simulink model "AircraftModelAdam"  (R2025b)
settings: Solver=VariableStepAuto  StartTime=0.0  StopTime=10  RelTol=1e-3
values from neighbouring files (symbols this model uses):
  forceConstants = [m; g]    [RunAircraftModel_AdamForceMomentVersion.m]
  maxAileronDeflection = 25*(pi/180)    (= 0.436332312999)    [RunAircraftModel_AdamForceMomentVersion.m]
  maxElevatorDeflection = 10*(pi/180)    (= 0.174532925199)    [RunAircraftModel_AdamForceMomentVersion.m]
  maxRudderDeflection = 30*(pi/180)    (= 0.523598775598)    [RunAircraftModel_AdamForceMomentVersion.m]
  momentConstants = [Jx; Jy; Jz; Jxz; Gamma]    [RunAircraftModel_AdamForceMomentVersion.m]
  U0 = 84.9905    [RunAircraftModel_AdamForceMomentVersion.m]
libraries: aerolibfltsims x2, aerolibanimutils x1
settings Model: Creator=Reza  LastModifiedBy=adaml
settings OptimizationCC: ReuseModelBlockBuffer=off
settings DebuggingCC: UnconnectedInputMsg=warning  UnconnectedOutputMsg=warning  UnconnectedLineMsg=warning
settings ModelReferenceCC: EnableRefExpFcnMdlSchedulingChecks=on
settings RTWCC: GPUComputeCapability=3.5  DLArmComputeVersion=19.05
settings SimscapeCC: SimscapeLogDecimation=1  SimscapeLogDataHistory=5000

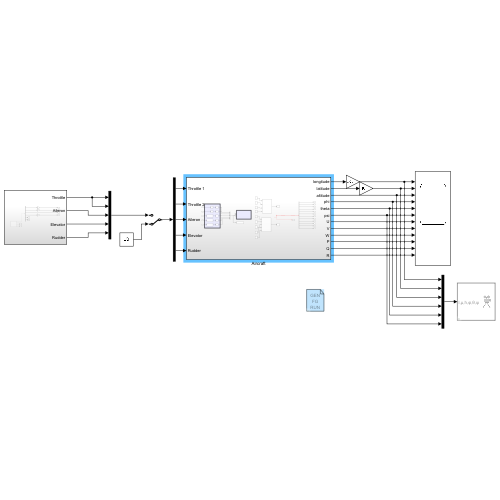
[thumbnail: Simulink's stored preview of the top-level diagram]
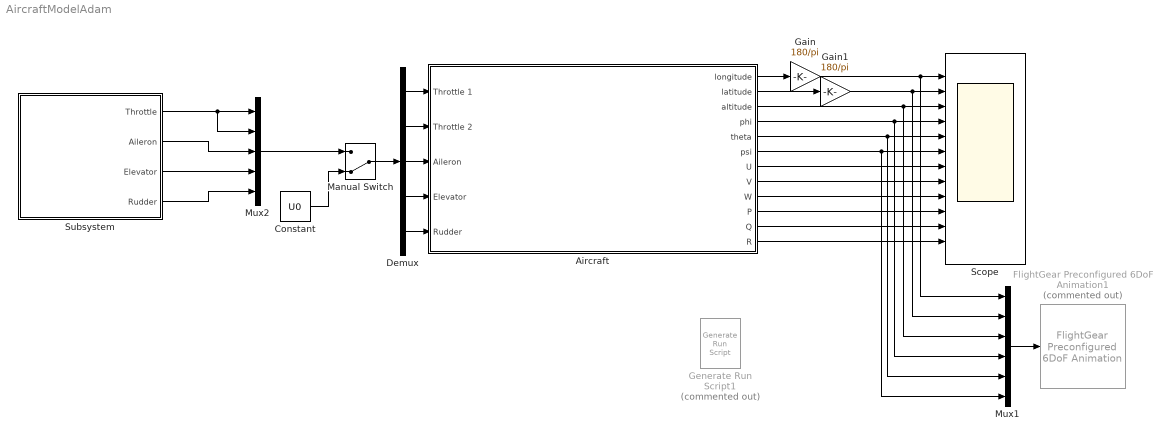
== system AircraftModelAdam ==
  Aircraft : Subsystem
  Constant : Constant  Value=U0
  Demux : Demux  Outputs=5
  FlightGear Preconfigured 6DoF Animation1 : aerolibfltsims/FlightGear Preconfigured 6DoF Animation  Commented=on  xFlightGearVersion=v2019.1  DestinationIpAddress=127.0.0.1  DestinationPort=5502  SampleTime=1/30  packetVersion=24
  Gain : Gain  Gain=180/pi
  Gain1 : Gain  Gain=180/pi
  Generate Run Script1 : aerolibfltsims/Generate Run Script  Commented=on  Architecture=Default  dataFlow=Send  GeometryModelName=b757  AirportId=YYZ  RunwayId=10L  InitialAltitude=7224  InitialHeading=0  OffsetDistance=4.72  OffsetAzimuth=0  InstallScenery=on  DisableShaders=on  OriginAddress=127.0.0.1  DestinationPort=5502  OriginPort=5505  LocalAddress=127.0.0.1  OutputFileName=runfg.bat  FlightGearBaseDirectory=C:\Program Files\FlightGear 2020.3
  Manual Switch : ManualSwitch  CurrentSetting=0
  Mux1 : Mux  Inputs=6
  Mux2 : Mux  Inputs=5
  Scope : Scope  NumInputPorts=12
      settings: ActiveDisplayYMinimum=-79.62713  ActiveDisplayYMaximum=-79.62453
  Subsystem : Subsystem
  wires:
  Constant/1 -> Manual Switch/2
  Mux2/1 -> Manual Switch/1
  Manual Switch/1 -> Demux/1
  Subsystem/1(Throttle) -> Mux2/2, Mux2/1
  Aircraft/7(U) -> Scope/7
  Aircraft/8(V) -> Scope/8
  Aircraft/9(W) -> Scope/9
  Aircraft/10(P) -> Scope/10
  Aircraft/11(Q) -> Scope/11
  Aircraft/12(R) -> Scope/12
  Demux/4 -> Aircraft/4(Elevator)
  Demux/1 -> Aircraft/1(Throttle 1)
  Demux/2 -> Aircraft/2(Throttle 2)
  Demux/3 -> Aircraft/3(Aileron)
  Demux/5 -> Aircraft/5(Rudder)
  Subsystem/2(Aileron) -> Mux2/3
  Subsystem/3(Elevator) -> Mux2/4
  Subsystem/4(Rudder) -> Mux2/5
  Aircraft/2(latitude) -> Gain1/1
  Aircraft/1(longitude) -> Gain/1
  Aircraft/4(phi) -> Mux1/4, Scope/4
  Aircraft/6(psi) -> Mux1/6, Scope/6
  Aircraft/3(altitude) -> Mux1/3, Scope/3
  Aircraft/5(theta) -> Mux1/5, Scope/5
  Mux1/1 -> FlightGear Preconfigured 6DoF Animation1/1
  Gain/1 -> Scope/1, Mux1/1
  Gain1/1 -> Scope/2, Mux1/2

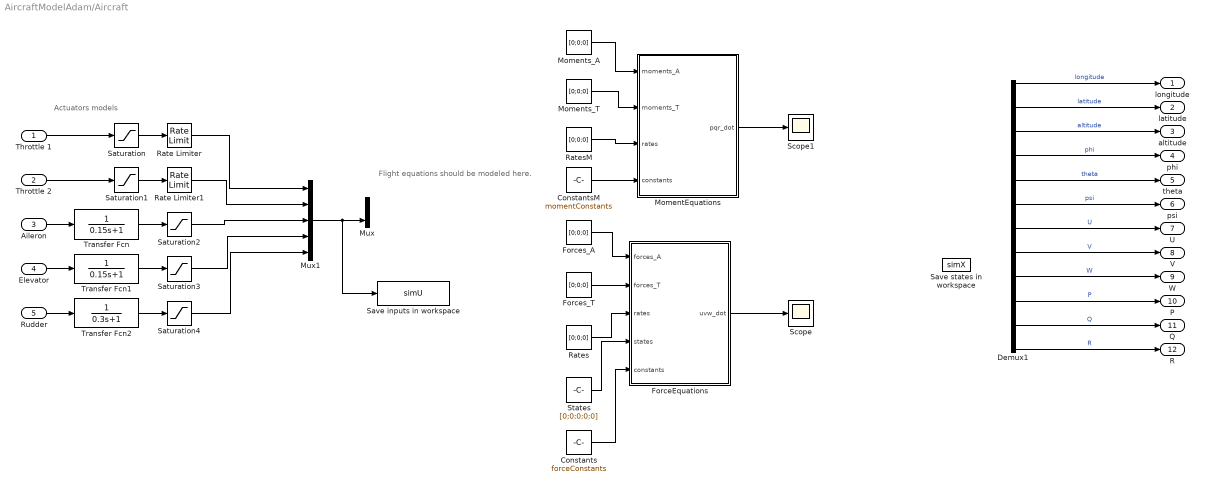
== system AircraftModelAdam/Aircraft ==
  note: Flight equations should be
      | modeled here.
  note: Actuators models
  Throttle 1 : Inport
  Throttle 2 : Inport  Port=2
  Aileron : Inport  Port=3
  Elevator : Inport  Port=4
  Rudder : Inport  Port=5
  Constants : Constant  Value=forceConstants
  ConstantsM : Constant  Value=momentConstants
  Demux1 : Demux  Outputs=12
  ForceEquations : MATLAB Function  TreatAsAtomicUnit=on
  Forces_A : Constant  Value=[0;0;0]
  Forces_T : Constant  Value=[0;0;0]
  MomentEquations : MATLAB Function  TreatAsAtomicUnit=on
  Moments_A : Constant  Value=[0;0;0]
  Moments_T : Constant  Value=[0;0;0]
  Mux : Mux  Inputs=2
  Mux1 : Mux  Inputs=5
  Rate Limiter : RateLimiter  RisingSlewLimit=1.6  FallingSlewLimit=-1.6  SampleTimeMode=inherited
  Rate Limiter1 : RateLimiter  RisingSlewLimit=1.6  FallingSlewLimit=-1.6  SampleTimeMode=inherited
  Rates : Constant  Value=[0;0;0]
  RatesM : Constant  Value=[0;0;0]
  Saturation : Saturate  UpperLimit=1  LowerLimit=0.5
  Saturation1 : Saturate  UpperLimit=1  LowerLimit=0.5
  Saturation2 : Saturate  UpperLimit=25*(pi/180)  LowerLimit=-25*(pi/180)
  Saturation3 : Saturate  UpperLimit=10*(pi/180)  LowerLimit=-10*(pi/180)
  Saturation4 : Saturate  UpperLimit=30*(pi/180)  LowerLimit=-30*(pi/180)
  Save inputs in workspace : ToWorkspace  VariableName=simU  SaveFormat=Timeseries  SampleTime=-1
  Save states in workspace : ToWorkspace  VariableName=simX  SaveFormat=Timeseries  SampleTime=-1
  Scope : Scope
      settings: ActiveDisplayYMinimum=-22.435878008720429  ActiveDisplayYMaximum=28.756040076197969
  Scope1 : Scope
      settings: ActiveDisplayYMinimum=-13.531899081321383  ActiveDisplayYMaximum=15.512627582639494  DataLoggingVariableName=ScopeData2
  States : Constant  Value=[0;0;0;0;0]
  Transfer Fcn : TransferFcn  Denominator=[0.15 1]
  Transfer Fcn1 : TransferFcn  Denominator=[0.15 1]
  Transfer Fcn2 : TransferFcn  Denominator=[0.3 1]
  longitude : Outport
  latitude : Outport  Port=2
  altitude : Outport  Port=3
  phi : Outport  Port=4
  theta : Outport  Port=5
  psi : Outport  Port=6
  U : Outport  Port=7
  V : Outport  Port=8
  W : Outport  Port=9
  P : Outport  Port=10
  Q : Outport  Port=11
  R : Outport  Port=12
  wires:
  ? -> Save states in workspace/1, Demux1/1
  Rate Limiter/1 -> Mux1/1
  Saturation4/1 -> Mux1/5
  Rate Limiter1/1 -> Mux1/2
  Demux1/6 -> psi/1  "psi"
  Saturation/1 -> Rate Limiter/1
  Mux1/1 -> Save inputs in workspace/1, Mux/2
  Demux1/2 -> latitude/1  "latitude"
  Demux1/10 -> P/1  "P"
  Aileron/1 -> Transfer Fcn/1
  Saturation2/1 -> Mux1/3
  Saturation3/1 -> Mux1/4
  Demux1/7 -> U/1  "U"
  Throttle 2/1 -> Saturation1/1
  Saturation1/1 -> Rate Limiter1/1
  Demux1/5 -> theta/1  "theta"
  Demux1/3 -> altitude/1  "altitude"
  Demux1/1 -> longitude/1  "longitude"
  Throttle 1/1 -> Saturation/1
  Elevator/1 -> Transfer Fcn1/1
  Rudder/1 -> Transfer Fcn2/1
  Demux1/4 -> phi/1  "phi"
  Demux1/9 -> W/1  "W"
  Demux1/11 -> Q/1  "Q"
  Demux1/12 -> R/1  "R"
  Demux1/8 -> V/1  "V"
  Transfer Fcn/1 -> Saturation2/1
  Transfer Fcn1/1 -> Saturation3/1
  Transfer Fcn2/1 -> Saturation4/1
  ForceEquations/1(uvw_dot) -> Scope/1
  Forces_A/1 -> ForceEquations/1(forces_A)
  Forces_T/1 -> ForceEquations/2(forces_T)
  Rates/1 -> ForceEquations/3(rates)
  States/1 -> ForceEquations/4(states)
  Constants/1 -> ForceEquations/5(constants)
  Moments_A/1 -> MomentEquations/1(moments_A)
  Moments_T/1 -> MomentEquations/2(moments_T)
  RatesM/1 -> MomentEquations/3(rates)
  ConstantsM/1 -> MomentEquations/4(constants)
  MomentEquations/1(pqr_dot) -> Scope1/1

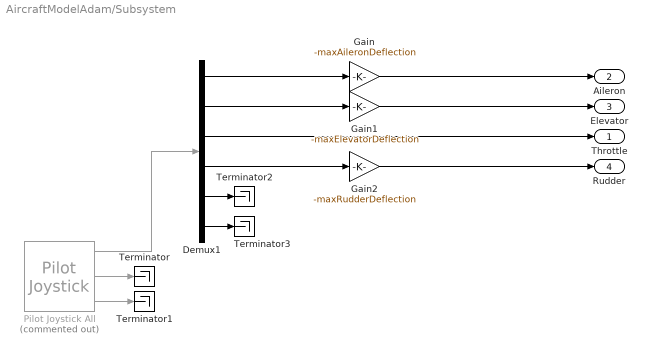
== system AircraftModelAdam/Subsystem ==
  Demux1 : Demux  Outputs=6
  Gain : Gain  Gain=-maxAileronDeflection
  Gain1 : Gain  Gain=-maxElevatorDeflection
  Gain2 : Gain  Gain=-maxRudderDeflection
  Pilot Joystick All : aerolibanimutils/Pilot Joystick  Commented=on  JoystickID=Joystick1  OutputConfiguration=AllOutputs  SampleTime=1/30
  Terminator{,1..3} (4 alike) : Terminator
  Throttle : Outport
  Aileron : Outport  Port=2
  Elevator : Outport  Port=3
  Rudder : Outport  Port=4
  wires:
  Demux1/3 -> Throttle/1
  Pilot Joystick All/3 -> Terminator1/1
  Demux1/4 -> Gain2/1
  Demux1/2 -> Gain1/1
  Pilot Joystick All/1 -> Demux1/1
  Demux1/5 -> Terminator2/1
  Demux1/6 -> Terminator3/1
  Pilot Joystick All/2 -> Terminator/1
  Demux1/1 -> Gain/1
  Gain/1 -> Aileron/1
  Gain1/1 -> Elevator/1
  Gain2/1 -> Rudder/1

== matlab function AircraftModelAdam/Aircraft/MomentEquations ==
  data: moments_A input; pqr_dot output; moments_T input; rates input; constants input
function pqr_dot = MomentEquations(moments_A, moments_T, rates, constants)
% moments_A = [lA; mA; nA]
% moments_T = [lT; mT; nT]
% rates     = [P; Q; R]
% constants = [Jx; Jy; Jz; Jxz; Gamma]

    lA = moments_A(1); mA = moments_A(2); nA = moments_A(3);
    lT = moments_T(1); mT = moments_T(2); nT = moments_T(3);

    P = rates(1); Q = rates(2); R = rates(3);

    Jx = constants(1);
    Jy = constants(2);
    Jz = constants(3);
    Jxz = constants(4);
    Gamma = constants(5);

    P_dot = (1/Gamma) * ...
        ( Jxz*(Jx - Jy + Jz)*P*Q ...
        - (Jz*(Jz - Jy) + Jxz^2)*Q*R ...
        + Jz*(lA + lT) ...
        + Jxz*(nA + nT) );

    Q_dot = (1/Jy) * ...
        ( (Jz - Jx)*P*R ...
        - Jxz*(P^2 - R^2) ...
        + (mA + mT) );

    R_dot = (1/Gamma) * ...
        ( ((Jx - Jy)*Jx + Jxz^2)*P*Q ...
        - Jxz*(Jx - Jy + Jz)*Q*R ...
        + Jxz*(lA + lT) ...
        + Jx*(nA + nT) );

    pqr_dot = [P_dot; Q_dot; R_dot];
end

== matlab function AircraftModelAdam/Aircraft/ForceEquations ==
  data: forces_A input; uvw_dot output; forces_T input; rates input; states input; constants input
function uvw_dot = ForceEquations(forces_A, forces_T, rates, states, constants)
% forces_A = [XA; YA; ZA]
% forces_T = [XT; YT; ZT]
% rates    = [P; Q; R]
% states   = [U; V; W; phi; theta]
% constants = [m; g]

    XA = forces_A(1); YA = forces_A(2); ZA = forces_A(3);
    XT = forces_T(1); YT = forces_T(2); ZT = forces_T(3);

    P = rates(1); Q = rates(2); R = rates(3);

    U = states(1); V = states(2); W = states(3);
    phi = states(4); theta = states(5);

    m = constants(1); g = constants(2);

    U_dot = R*V - Q*W - g*sin(theta) + (XT + XA)/m;
    V_dot = -R*U + P*W + g*sin(phi)*cos(theta) + (YT + YA)/m;
    W_dot = Q*U - P*V + g*cos(phi)*cos(theta) + (ZT + ZA)/m;

    uvw_dot = [U_dot; V_dot; W_dot];
end
